simulink model "eAgriBot_V4"  (R2022b)
settings: Solver=ode3  StartTime=0.0  StopTime=t_sim  FixedStep=step_size  RelTol=1e-3
values from neighbouring files (symbols this model uses):
  accel = 0.1*9.81    (= 0.981)    [Run_eAgriBot_V4.m]
  B_tines = 5    [Run_eAgriBot_V4.m]
  brake_bias = 1    [Run_eAgriBot_V4.m]
  c = 6100    [Run_eAgriBot_V4.m]
  decel = 0.15*9.81    (= 1.4715)    [Run_eAgriBot_V4.m]
  decel_begin_dist = total_dist_target    (= 100)    [Run_eAgriBot_V4.m]
  drivetype = 3    [Run_eAgriBot_V4.m]
  effmap = [0.5 0.586 0.723 0.778 0.614 0.604 0.6 0.584 0.709 0.658 0.586 0.688 ... (121 elements, 11x11)]    [EM_effmap_generic.mat]
  end_delay = 4    [Run_eAgriBot_V4.m]
  F_tines = 5    [Run_eAgriBot_V4.m]
  Fb_max = m*g    (= 5101.2)    [Run_eAgriBot_V4.m]
  FT_c_x_rel = l_f    (= 0.645)    [Run_eAgriBot_V4.m]
  FT_c_z_rel = R_u-h_CoG    (= -0.2825)    [Run_eAgriBot_V4.m]
  g = 9.81    [Run_eAgriBot_V4.m]
  gb_eff = 0.98    [Run_eAgriBot_V4.m]
  ground_coh = c*ones(length(ground_points),1)    [Run_eAgriBot_V4.m]
  ground_dens = gamma_s*ones(length(ground_points),1)    [Run_eAgriBot_V4.m]
  ground_height = zeros(length(ground_points),1)    [Run_eAgriBot_V4.m]
  ground_kxy = k_xy*ones(length(ground_points),1)    [Run_eAgriBot_V4.m]
  ground_res = 0.01    [Run_eAgriBot_V4.m]
  Har_back_tip_x_rel = Har_back_top_x_rel+Har_tine_length*cos(Har_angle)    [Run_eAgriBot_V4.m]
  Har_back_tip_z_rel = abs(Hook_z_rel)-h_CoG-Har_tine_depth    [Run_eAgriBot_V4.m]
  Har_back_top_x_rel = -2.0    (= -2)    [Run_eAgriBot_V4.m]
  Har_back_top_z_rel = Har_back_tip_z_rel+Har_tine_length*sin(Har_angle)    [Run_eAgriBot_V4.m]
  Har_front_tip_x_rel = Har_front_top_x_rel+Har_tine_length*cos(Har_angle)    [Run_eAgriBot_V4.m]
  Har_front_tip_z_rel = abs(Hook_z_rel)-h_CoG-Har_tine_depth    [Run_eAgriBot_V4.m]
  Har_front_top_x_rel = -1.2    [Run_eAgriBot_V4.m]
  Har_front_top_z_rel = Har_front_tip_z_rel+Har_tine_length*sin(Har_angle)    [Run_eAgriBot_V4.m]
  Har_tine_length = 0.25    [Run_eAgriBot_V4.m]
  Har_tine_width = 0.02    [Run_eAgriBot_V4.m]
  Har_tire_rad = 0.5842/2    (= 0.2921)    [Run_eAgriBot_V4.m]
  Har_tire_x_rel = -1.5    [Run_eAgriBot_V4.m]
  Har_tire_z_rel = abs(Hook_z_rel)-h_CoG+Har_tire_rad    [Run_eAgriBot_V4.m]
  Hook_x_rel = l_f-l-0.4    (= -1.045)    [Run_eAgriBot_V4.m]
  Hook_z_rel = -0.3    [Run_eAgriBot_V4.m]
  i_front = 17.9542    [Run_eAgriBot_V4.m]
  I_gain = 0.0    (= 0)    [Run_eAgriBot_V4.m]
  i_rear = 17.9542    [Run_eAgriBot_V4.m]
  I_y = 150    [Run_eAgriBot_V4.m]
  I_y_tool = 20    [Run_eAgriBot_V4.m]
  index_init = round(FT_init_exit_x/ground_res)+1    [Run_eAgriBot_V4.m]
  init_CoG_height = h_CoG-0.001    (= 0.599)    [Run_eAgriBot_V4.m]
  init_CoG_v_z = 0    [Run_eAgriBot_V4.m]
  init_omega = 0    [Run_eAgriBot_V4.m]
  init_theta = 0    [Run_eAgriBot_V4.m]
  J_front = J_drive    (= 15)    [Run_eAgriBot_V4.m]
  J_harrow = 1    [Run_eAgriBot_V4.m]
  J_rear = J_drive    (= 15)    [Run_eAgriBot_V4.m]
  k_d = 50e2    (= 5000)    [Run_eAgriBot_V4.m]
  k_d_har = 50e2    (= 5000)    [Run_eAgriBot_V4.m]
  m = 520    [Run_eAgriBot_V4.m]
  m_tool = 200    [Run_eAgriBot_V4.m]
  main_cycle_delay = 5    [Run_eAgriBot_V4.m]
  mu = 0.35    [Run_eAgriBot_V4.m]
  omega_tool_init = 0    [Run_eAgriBot_V4.m]
  P_aux = 200    [Run_eAgriBot_V4.m]
  P_gain = 1.0    (= 1)    [Run_eAgriBot_V4.m]
  pack_Ah = 360    [Battery_data_V5_Kokam_NMC.mat]
  pack_R_charge = [0.00267222222222 0.00267222222222 0.00317777777778 0.00310555555556 0.0026 0.00281666666667 0.00332222222222 0.00353888888889 0.00325 0.00382777777778 0.00382777777778]    [Battery_data_V5_Kokam_NMC.mat]
  pack_R_discharge = [0.00267222222222 0.00267222222222 0.00317777777778 0.00310555555556 0.0026 0.00281666666667 0.00332222222222 0.00353888888889 0.00325 0.00382777777778 0.00382777777778]    [Battery_data_V5_Kokam_NMC.mat]
  pack_VOC = [54.509 52.351 50.895 49.556 48.477 47.645 47.008 46.449 45.825 44.941 44.941]    [Battery_data_V5_Kokam_NMC.mat]
  params2 = [exit_angle reso theta_m_max s_d_tol po]    [Run_eAgriBot_V4.m]
  phi = 26.6    [Run_eAgriBot_V4.m]
  pre_accel = 0.1*9.81    (= 0.981)    [Run_eAgriBot_V4.m]
  pre_decel = 0.15*9.81    (= 1.4715)    [Run_eAgriBot_V4.m]
  pre_decel_begin_dist = pre_dist_target-pre_decel_dist    (= 2.34454218631)    [Run_eAgriBot_V4.m]
  pre_vel = 5    [Run_eAgriBot_V4.m]
  r_front = R_u    (= 0.3175)    [Run_eAgriBot_V4.m]
  r_rear = R_u    (= 0.3175)    [Run_eAgriBot_V4.m]
  rho_t = gamma_s/9.81    (= 1664.01630989)    [Run_eAgriBot_V4.m]
  RT_c_x_rel = l_f-l    (= -0.645)    [Run_eAgriBot_V4.m]
  RT_c_z_rel = R_u-h_CoG    (= -0.2825)    [Run_eAgriBot_V4.m]
  s_init = 3    [Run_eAgriBot_V4.m]
  simu_max_time = cycle_total_time*4    (= 259.930519878)    [Run_eAgriBot_V4.m]
  slip_init = 0    [Run_eAgriBot_V4.m]
  slip_ub = r_rear*1.75    (= 0.555625)    [Run_eAgriBot_V4.m]
  slip_ub_har = Har_tire_rad*1.90    (= 0.55499)    [Run_eAgriBot_V4.m]
  SOC_init = 0.8    [Run_eAgriBot_V4.m]
  SOD = [0 0.1 0.2 0.3 0.4 0.5 0.6 0.7 0.8 0.9 1]    [Battery_data_V5_Kokam_NMC.mat]
  sr_lim_skid = -0.2    [Run_eAgriBot_V4.m]
  sr_lim_slip_f = 0.20-slip_trig    (= 0.18)    [Run_eAgriBot_V4.m]
  sr_lim_slip_r = 0.14-slip_trig    (= 0.12)    [Run_eAgriBot_V4.m]
  step_size = 1e-3    (= 0.001)    [Run_eAgriBot_V4.m]
  T = [80 80 75 70.5882352941 66.6666666667 63.1578947368 60 57.1428571429 54.5454545455 52.1739130435 50 48 ... (49 elements, 49x1)]    [EM_data_V4.mat]    (also in Run_eAgriBot_V4.m = 2*T)
  T_effmap = [0 8 16 24 32 40 48 56 64 72 80]    [EM_effmap_generic.mat]    (also in Run_eAgriBot_V4.m = 2*T_effmap)
  T_multi_r = 1.5    [Run_eAgriBot_V4.m]
  t_params = [c k_c k_phi phi k_xy gamma_s R_u wid c_0 c_1 c_0f c_1f n_0 n_1 k_1 k_2 k_3]    [Run_eAgriBot_V4.m]
  t_params_har = [c k_c k_phi phi k_xy gamma_s Har_tire_rad Har_tire_wid c_0 c_1 c_0f c_1f n_0 n_1 k_1 k_2 k_3]    [Run_eAgriBot_V4.m]
  theta_tool_init = 0    [Run_eAgriBot_V4.m]
  Tine_vz_damping = 0    [Run_eAgriBot_V4.m]
  Tool_x_rel = -1.3    [Run_eAgriBot_V4.m]
  Tool_z_rel = -0.08    [Run_eAgriBot_V4.m]
  v_init = 0    [Run_eAgriBot_V4.m]
  vel_max = 8    [Run_eAgriBot_V4.m]
  w = [0 75 80 85 90 95 100 105 110 115 120 125 ... (49 elements, 49x1)]    [EM_data_V4.mat]
  w_effmap = [0 31.4159265359 62.8318530718 94.2477796077 125.663706144 157.079632679 188.495559215 219.911485751 251.327412287 282.743338823 314.159265359]    [EM_effmap_generic.mat]
libraries: slpidlib x1, simulink x1
(part 3 of 4)

== system eAgriBot_V4/Vehicle dynamics/Towed tool calculations/Vertical force damping ==
  Har_tire_z : Inport
  Har_tire_vz : Inport  Port=2
  F_sigma_zhar : Inport  Port=3
  F_tau_zhar : Inport  Port=4
  Abs : Abs  SaturateOnIntegerOverflow=off
  Abs1 : Abs  SaturateOnIntegerOverflow=off
  Constant2 : Constant  Value=0
  Constant3 : Constant  Value=0
  Constant4 : Constant  Value=0
  Divide : Product  Inputs=*/
  Divide1 : Product  Inputs=*/
  Gain2 : Gain  Gain=k_d_har
  Product : Product
  Product1 : Product
  Sum1 : Sum  Inputs=|+-
  Sum2 : Sum  Inputs=|++
  Sum3 : Sum  Inputs=|++
  Sum4 : Sum  Inputs=-+|
  Sum5 : Sum  Inputs=|++
  Switch2 : Switch  Criteria=u2 > Threshold  SaturateOnIntegerOverflow=off  InputSameDT=off
  Switch3 : Switch  Criteria=u2 ~= 0  SaturateOnIntegerOverflow=off  InputSameDT=off
  Switch4 : Switch  Criteria=u2 ~= 0  SaturateOnIntegerOverflow=off  InputSameDT=off
  To Workspace1 : ToWorkspace  VariableName=Fz_har  SaveFormat=Timeseries  SampleTime=-1
  F_sigma_zhar_d : Outport
  F_tau_zhar_d : Outport  Port=2
  wires:
  Sum1/1 -> Sum5/1, F_sigma_zhar_d/1
  Har_tire_vz/1 -> Gain2/1
  Gain2/1 -> Switch2/3
  Har_tire_z/1 -> Switch2/2
  Switch2/1 -> Product1/1, Product/1
  Constant2/1 -> Switch2/1
  Sum2/1 -> Divide/2, Switch3/2
  Constant3/1 -> Switch3/3
  Divide/1 -> Abs/1
  Abs/1 -> Switch3/1
  Switch3/1 -> Product/2
  Product/1 -> Sum1/2
  Sum3/1 -> Divide1/2, Switch4/2
  Abs1/1 -> Switch4/1
  Constant4/1 -> Switch4/3
  F_tau_zhar/1 -> Sum4/2, Sum3/1, Divide1/1, Sum2/2
  Divide1/1 -> Abs1/1
  F_sigma_zhar/1 -> Sum2/1, Sum3/2, Sum1/1, Divide/1
  Switch4/1 -> Product1/2
  Product1/1 -> Sum4/1
  Sum4/1 -> Sum5/2, F_tau_zhar_d/1
  Sum5/1 -> To Workspace1/1

== system eAgriBot_V4/Vehicle dynamics/Towed tool calculations/Vertical force damping1 ==
  Har_tire_z : Inport
  Har_tire_vz : Inport  Port=2
  F_sigma_zhar : Inport  Port=3
  Constant2 : Constant  Value=0
  Gain2 : Gain  Gain=k_d_har
  Sum1 : Sum  Inputs=|+-
  Switch2 : Switch  Criteria=u2 > Threshold  SaturateOnIntegerOverflow=off  InputSameDT=off
  F_sigma_zhar_d : Outport
  wires:
  Sum1/1 -> F_sigma_zhar_d/1
  Har_tire_vz/1 -> Gain2/1
  Gain2/1 -> Switch2/3
  Har_tire_z/1 -> Switch2/2
  Switch2/1 -> Sum1/2
  Constant2/1 -> Switch2/1
  F_sigma_zhar/1 -> Sum1/1

== matlab function eAgriBot_V4/Vehicle dynamics/Position and velocity of the wheels (output values are for wheel bottom points)/MATLAB Function ==
  data: theta input; RT_x output; RT_z output; FT_x output; FT_z output; RT_vx output; RT_vz output; FT_vx output; FT_vz output; omega input; CoG_vx input; CoG_x input; CoG_vz input; CoG_z input; RT_c_z_rel input; RT_c_x_rel input; FT_c_z_rel input; FT_c_x_rel input; r_rear input; r_front input
function [RT_x, RT_z, FT_x, FT_z, RT_vx, RT_vz, FT_vx, FT_vz] =...
    fcn(theta, omega, CoG_vx, CoG_x, CoG_vz, CoG_z, RT_c_z_rel,...
    RT_c_x_rel, FT_c_z_rel, FT_c_x_rel, r_rear, r_front)

    % theta: Vehicle pitch
    % omega: Vehicle pitch rate
    % CoG_x: Current x-position of the CoG
    % CoG_z: Current z-position of the CoG
    % RT/FT_c_z_rel: Difference between rear/front tire z-coordinate and the CoG
    % z-coordinate when pitch is zero.
    % RT/FT_c_x_rel: Difference between rear/front tire x-coordinate and the CoG
    % x-coordinate when pitch is zero.
    % r_rear: Rear tire radius
    % r_front: Front tire radius
    
    RT_center = [cos(theta) sin(theta); -sin(theta) cos(theta)]*...
        [RT_c_x_rel; RT_c_z_rel]+[CoG_x; CoG_z];
    
    RT_x = RT_center(1);
    RT_z = RT_center(2)-r_rear;
    
    FT_center = [cos(theta) sin(theta); -sin(theta) cos(theta)]*...
        [FT_c_x_rel; FT_c_z_rel]+[CoG_x; CoG_z];
    
    FT_x = FT_center(1);
    FT_z = FT_center(2)-r_front;
    
    RT_vec_x = RT_x-CoG_x;
    RT_vec_z = RT_z-CoG_z;
    RT_vec = [RT_vec_x; 0; RT_vec_z];
    
    RT_vel = [CoG_vx; 0; CoG_vz]+cross([0; omega; 0], RT_vec);
    RT_vx = RT_vel(1);
    RT_vz = RT_vel(3);
    
    FT_vec_x = FT_x-CoG_x;
    FT_vec_z = FT_z-CoG_z;
    FT_vec = [FT_vec_x; 0; FT_vec_z];
    
    FT_vel = [CoG_vx; 0; CoG_vz]+cross([0; omega; 0], FT_vec);
    FT_vx = FT_vel(1);
    FT_vz = FT_vel(3);

end

== matlab function eAgriBot_V4/Vehicle dynamics/Ground properties update for rear tire/MATLAB Function ==
  data: index_upd_high output; index_upd_low output; t_params input; ground_res input; ground_height output; dens output; coh output; kx output; params2 input; FT_x input; FT_z input; sr_f input; ground_height input; dens input; coh input; kx input; prev_index input; index output
function [index_upd_high, index_upd_low, ground_height, dens, coh, kx, index]= fcn(t_params, ground_res, params2,...
    FT_x, FT_z, sr_f, ground_height, dens, coh, kx, prev_index)

    R_u = t_params(7);
    ea = deg2rad(params2(1));
    c = t_params(1);
    gamma_s = t_params(6);
    k_x = t_params(5);
    k_1 = t_params(15);
    k_2 = t_params(16);
    k_3 = t_params(17);

    n_p = 1;

    FT_exit_x = FT_x+R_u*sin(ea);
    FT_exit_z = FT_z+(R_u-R_u*cos(ea));

    FT_exit_dens = gamma_s*(1+(1-exp(-abs(sr_f)/k_1))*k_2+k_3*n_p);
    FT_exit_coh = c*(1+(1-exp(-abs(sr_f)/k_1))*k_2+k_3*n_p);
    FT_exit_kx = k_x*(1-(1-exp(-abs(sr_f)/k_1))*k_2-k_3*n_p);

    index = round(FT_exit_x/ground_res)+1;

    ground_height(index,1) = FT_exit_z;

    dens(index,1) = FT_exit_dens;

    coh(index,1) = FT_exit_coh;

    kx(index,1) = FT_exit_kx;
    
    % index_upd_high and index_upd_low are needed for updating the soil
    % values for the harrow tines
    index_upd_high = index;
    index_upd_low = index;


    if index > (prev_index+1)
        num_points_tofix = index-(prev_index+1);
        index_upd_low = prev_index+1;
        for i = 1:num_points_tofix
            ground_height(prev_index+i,1) = (ground_height(index,1)-ground_height(prev_index,1))*...
                i/(num_points_tofix+1)+ground_height(prev_index,1);

            dens(prev_index+i,1) = (dens(index,1)-dens(prev_index,1))*...
                i/(num_points_tofix+1)+dens(prev_index,1);

            coh(prev_index+i,1) = (coh(index,1)-coh(prev_index,1))*...
                i/(num_points_tofix+1)+coh(prev_index,1);

            kx(prev_index+i,1) = (kx(index,1)-kx(prev_index,1))*...
                i/(num_points_tofix+1)+kx(prev_index,1);
        end
    end

end

== matlab function eAgriBot_V4/Vehicle dynamics/Ground properties update for rear tire/MATLAB Function1 ==
  data: RT_x input; RT_z input; ground_height input; dens input; coh input; kx input; ground_res input; t_params input; upd_RT_z output; upd_dens output; upd_coh output; upd_kx output
function [upd_RT_z, upd_dens, upd_coh, upd_kx] = fcn(RT_x, RT_z, ground_height, dens, coh, kx, ground_res, t_params)

    
    R_u = t_params(7);
    ind_L = max(round((RT_x-R_u)/ground_res)+1, 1);
    ind_R = max(round((RT_x+R_u)/ground_res)+1, 1);

    upd_RT_z = RT_z-mean(ground_height(ind_L:ind_R));
    upd_dens = mean(dens(ind_L:ind_R));
    upd_coh = mean(coh(ind_L:ind_R));
    upd_kx = mean(kx(ind_L:ind_R));

end

== matlab function eAgriBot_V4/Vehicle dynamics/Towed tool calculations/Tool position, velocity, and acceleration calc/Tool position, velocity, and acceleration calc ==
  data: alpha input; omega input; theta input; Hook_x output; CoG_x input; CoG_z input; CoG_v_x input; CoG_v_z input; CoG_a_x input; CoG_a_z input; alpha_tool input; omega_tool input; theta_tool input; Hook_x_rel input; Hook_z_rel input; Hook_z output; Hook_v_x output; Hook_v_z output; Hook_a_x output; Hook_a_z output; Tool_CoG_x output; Tool_CoG_z output; Tool_CoG_a_x output; Tool_CoG_a_z output; Tool_x_rel input; Tool_z_rel input; Har_back_top_x_rel input; Har_back_top_z_rel input; Har_back_tip_x_rel input; Har_back_tip_z_rel input; Har_front_top_x_rel input; Har_front_top_z_rel input; Har_front_tip_x_rel input; Har_front_tip_z_rel input; Har_tire_x_rel input; Har_tire_z_rel input; Har_tire_radius input; Harrow_back_mid_x output; Harrow_back_mid_z output; Harrow_back_tip_z output; Harrow_back_mid_v_x output; Harrow_back_mid_v_z output; Harrow_front_mid_x output; Harrow_front_mid_z output; Harrow_front_tip_z output; Harrow_front_mid_v_x output; Harrow_front_mid_v_z output; Harrow_tire_bottom_x output; Harrow_tire_bottom_z output; Harrow_tire_bottom_v_x output; Harrow_tire_bottom_v_z output; Harrow_back_angle output; Harrow_front_angle output; Harrow_front_tip_x output; Harrow_back_tip_x output
function [Hook_x, Hook_z, Hook_v_x, Hook_v_z, Hook_a_x, Hook_a_z,...
    Tool_CoG_x, Tool_CoG_z, Tool_CoG_a_x, Tool_CoG_a_z,...
    Harrow_back_mid_x,...
    Harrow_back_mid_z, Harrow_back_tip_z, Harrow_back_mid_v_x,...
    Harrow_back_mid_v_z, Harrow_front_mid_x, Harrow_front_mid_z,...
    Harrow_front_tip_z, Harrow_front_mid_v_x, Harrow_front_mid_v_z,...
    Harrow_tire_bottom_x, Harrow_tire_bottom_z, Harrow_tire_bottom_v_x,...
    Harrow_tire_bottom_v_z, Harrow_back_angle, Harrow_front_angle, Harrow_front_tip_x,...
    Harrow_back_tip_x] = fcn(alpha,...
    omega, theta, CoG_x, CoG_z, CoG_v_x, CoG_v_z, CoG_a_x, CoG_a_z, alpha_tool,...
    omega_tool, theta_tool, Hook_x_rel, Hook_z_rel, Tool_x_rel, Tool_z_rel,...
    Har_back_top_x_rel, Har_back_top_z_rel,...
    Har_back_tip_x_rel, Har_back_tip_z_rel, Har_front_top_x_rel, Har_front_top_z_rel,...
    Har_front_tip_x_rel, Har_front_tip_z_rel, Har_tire_x_rel, Har_tire_z_rel, Har_tire_radius)

    % Calculate the current position of the hook

    % Hook_x_rel and Hook_z_rel describe the position of the hook in
    % relation to the CoG of the vehicle when the vehicle is on flat
    % ground.
    Hook_pos = [cos(theta) sin(theta); -sin(theta) cos(theta)]*...
            [Hook_x_rel; Hook_z_rel]+[CoG_x; CoG_z];
    
    Hook_x = Hook_pos(1);
    Hook_z = Hook_pos(2);

    % Calculate the current velocity of the hook
    vec_CoG_hook = [Hook_x-CoG_x; 0; Hook_z-CoG_z];
    Hook_v = [CoG_v_x; 0; CoG_v_z] + cross([0; omega; 0], vec_CoG_hook);

    Hook_v_x = Hook_v(1);
    Hook_v_z = Hook_v(3);

    % Calculate the current acceleration of the hook

    alpha_2 = [0; alpha; 0];
    omega_2 = [0; omega; 0];

    Hook_a = [CoG_a_x; 0; CoG_a_z] + cross(alpha_2, vec_CoG_hook) + cross(omega_2, cross(omega_2, vec_CoG_hook));

    Hook_a_x = Hook_a(1);
    Hook_a_z = Hook_a(3);

    % Calculate the current acceleration of the CoG of the tool

    % Tool_x_rel and Tool_z_rel describe the position of the tool CoG in
    % relation to the hook when the vehicle is on flat
    % ground.
    Tool_CoG_pos = [cos(theta_tool) sin(theta_tool); -sin(theta_tool) cos(theta_tool)]*...
            [Tool_x_rel; Tool_z_rel]+[Hook_x; Hook_z];

    Tool_CoG_x = Tool_CoG_pos(1);
    Tool_CoG_z = Tool_CoG_pos(2);

    vec_toolCoG_hook = [Hook_x-Tool_CoG_x; 0; Hook_z-Tool_CoG_z];

    alpha_tool_2 = [0; alpha_tool; 0];
    omega_tool_2 = [0; omega_tool; 0];

    Tool_CoG_a = Hook_a - cross(alpha_tool_2,vec_toolCoG_hook) - cross(omega_tool_2, cross(omega_tool_2,vec_toolCoG_hook));

    Tool_CoG_a_x = Tool_CoG_a(1);
    Tool_CoG_a_z = Tool_CoG_a(3);

    % Calculate the current position and velocity of the bottom point of
    % the tool.

    % Tool_bottom_x_rel and Tool_bottom_z_rel describe the position of the
    % bottom point of the tool in relation to the hook when the vehicle and
    % tool are on flat ground.

    % New stuff, harrow

    Harrow_back_top_pos = [cos(theta_tool) sin(theta_tool); -sin(theta_tool) cos(theta_tool)]*...
        [Har_back_top_x_rel; Har_back_top_z_rel]+[Hook_x; Hook_z];
    
    Harrow_back_tip_pos = [cos(theta_tool) sin(theta_tool); -sin(theta_tool) cos(theta_tool)]*...
        [Har_back_tip_x_rel; Har_back_tip_z_rel]+[Hook_x; Hook_z];

    Harrow_back_tip_x = Harrow_back_tip_pos(1);
    Harrow_back_tip_z = Harrow_back_tip_pos(2);

    Harrow_front_top_pos = [cos(theta_tool) sin(theta_tool); -sin(theta_tool) cos(theta_tool)]*...
        [Har_front_top_x_rel; Har_front_top_z_rel]+[Hook_x; Hook_z];

    Harrow_front_tip_pos = [cos(theta_tool) sin(theta_tool); -sin(theta_tool) cos(theta_tool)]*...
        [Har_front_tip_x_rel; Har_front_tip_z_rel]+[Hook_x; Hook_z];

    Harrow_front_tip_x = Harrow_front_tip_pos(1);
    Harrow_front_tip_z = Harrow_front_tip_pos(2);

    % Back row
    
    if Harrow_back_top_pos(2) >= 0
        Harrow_back_mid_z = Harrow_back_tip_pos(2)/2;
        % Calculate gradient and constant (c) in line equation
        Harrow_back_grad = (Harrow_back_tip_pos(2)-Harrow_back_top_pos(2))/(Harrow_back_tip_pos(1)-Harrow_back_top_pos(1));
        Harrow_back_c = Harrow_back_tip_pos(2)-Harrow_back_tip_pos(1)*Harrow_back_grad;
        % Calculate mid point of the tine
        Harrow_back_mid_x = (Harrow_back_mid_z-Harrow_back_c)/Harrow_back_grad;
    else
        Harrow_back_mid_z = (Harrow_back_tip_pos(2)+Harrow_back_top_pos(2))/2;
        Harrow_back_mid_x = (Harrow_back_tip_pos(1)+Harrow_back_top_pos(1))/2;
    end
    Harrow_back_angle = -1*asin((Harrow_back_tip_pos(2)-Harrow_back_top_pos(2))/(Harrow_back_tip_pos(1)-Harrow_back_top_pos(1)));
    Harrow_back_depth = Harrow_back_tip_pos(2);

    vec_Hook_backtip = [Harrow_back_tip_pos(1)-Hook_x; 0; Harrow_back_tip_pos(2)-Hook_z];
    Harrow_back_mid_v = [Hook_v_x; 0; Hook_v_z] + cross([0; omega_tool; 0], vec_Hook_backtip);

    Harrow_back_mid_v_x = Harrow_back_mid_v(1);
    Harrow_back_mid_v_z = Harrow_back_mid_v(3);

    % Front row
    
    if Harrow_front_top_pos(2) >= 0
        Harrow_front_mid_z = Harrow_front_tip_pos(2)/2;
        % Calculate gradient and constant (c) in line equation
        Harrow_front_grad = (Harrow_front_tip_pos(2)-Harrow_front_top_pos(2))/(Harrow_front_tip_pos(1)-Harrow_front_top_pos(1));
        Harrow_front_c = Harrow_front_tip_pos(2)-Harrow_front_tip_pos(1)*Harrow_front_grad;
        % Calculate mid point of the tine
        Harrow_front_mid_x = (Harrow_front_mid_z-Harrow_front_c)/Harrow_front_grad;
    else
        Harrow_front_mid_z = (Harrow_front_tip_pos(2)+Harrow_front_top_pos(2))/2;
        Harrow_front_mid_x = (Harrow_front_tip_pos(1)+Harrow_front_top_pos(1))/2;
    end
    Harrow_front_angle = -1*asin((Harrow_front_tip_pos(2)-Harrow_front_top_pos(2))/(Harrow_front_tip_pos(1)-Harrow_front_top_pos(1)));
    Harrow_front_depth = Harrow_front_tip_pos(2);

    vec_Hook_fronttip = [Harrow_front_tip_pos(1)-Hook_x; 0; Harrow_front_tip_pos(2)-Hook_z];
    Harrow_front_mid_v = [Hook_v_x; 0; Hook_v_z] + cross([0; omega_tool; 0], vec_Hook_fronttip);

    Harrow_front_mid_v_x = Harrow_front_mid_v(1);
    Harrow_front_mid_v_z = Harrow_front_mid_v(3);

    Harrow_tire_pos = [cos(theta_tool) sin(theta_tool); -sin(theta_tool) cos(theta_tool)]*...
        [Har_tire_x_rel; Har_tire_z_rel]+[Hook_x; Hook_z];

    Harrow_tire_bottom_x = Harrow_tire_pos(1);
    Harrow_tire_bottom_z = Harrow_tire_pos(2)-Har_tire_radius;
    
    vec_Hook_tirebottom = [Harrow_tire_bottom_x-Hook_x; 0; Harrow_tire_bottom_z-Hook_z];
    Harrow_tire_bottom_v = [Hook_v_x; 0; Hook_v_z] + cross([0; omega_tool; 0], vec_Hook_tirebottom);

    Harrow_tire_bottom_v_x = Harrow_tire_bottom_v(1);
    Harrow_tire_bottom_v_z = Harrow_tire_bottom_v(3);

    % Needs to output:
    % Harrow_back_mid_x, Harrow_back_mid_z, Harrow_back_tip_z
    % Harrow_back_mid_v_x, Harrow_back_mid_v_z
    % Harrow_front_mid_x, Harrow_front_mid_z, Harrow_front_tip_z
    % Harrow_front_mid_v_x, Harrow_front_mid_v_z
    % Harrow_tire_bottom_x, Harrow_tire_bottom_z
    % Harrow_tire_bottom_v_x, Harrow_tire_bottom_v_z

    % Needs as inputs:
    % Har_back_top_x_rel, Har_back_top_z_rel
    % Har_back_tip_x_rel, Har_back_tip_z_rel
    % Har_front_top_x_rel, Har_front_top_z_rel
    % Har_front_tip_x_rel, Har_front_tip_z_rel
    % Har_tire_x_rel, Har_tire_z_rel, Har_tire_radius

end

== matlab function eAgriBot_V4/Tire model (FRONT)/slip_ratio calc ==
  data: r_front input; v_ms input; FT_vx input; w_tire input; sr output; slip_ub input
function sr = fcn(r_front, v_ms, FT_vx, w_tire, slip_ub)
    
    ub = slip_ub; % upper bound (when the rotational speed is 1 rad/s)
    lb = 0.1/3.6; % lower bound

    v_ms = max(0, v_ms);

    if abs(v_ms) > ub
        sr = (w_tire*r_front-FT_vx)/FT_vx;
    elseif abs(v_ms) < lb
        sr = w_tire*r_front-FT_vx;
    elseif abs(v_ms) <= ub && abs(v_ms) >= lb
        sr = (1/(ub-lb))*(ub-v_ms)*(w_tire*r_front-FT_vx)+(1/(ub-lb))*(v_ms-lb)*((w_tire*r_front-FT_vx)/FT_vx);
    else
        sr = 0;
    end
    
    sr = max(-1, sr);

end

== matlab function eAgriBot_V4/Tire model (REAR)/Tire force calc1 ==
  data: T output; v_ms input; w_tire_pure input; s_d input; t_params input; params2 input; h input; gamma_s input; c input; k_xy input; F_sigma_z output; F_sigma_x output; F_sigma_angle output; F_tau_z output; F_tau_x output; F_tau_angle output; drivetype input
function [T, F_sigma_z, F_sigma_x, F_sigma_angle, F_tau_z, F_tau_x, F_tau_angle]  = fcn(v_ms, w_tire_pure, s_d, t_params, params2, h, gamma_s, c, k_xy, drivetype)

    %%

% function [W, F_x, T] = ReeceFuncSim_V1(s_d, h, t_params, params2)
%     c = t_params(1); % Pa
    k_c = t_params(2); % 34 default
    k_phi = t_params(3); % 49.68 default
    % n = 0.7;
    phi = t_params(4); % deg
%     k_xy = t_params(5); % m
%     gamma_s = t_params(6); % N/m^3
    
    R_u = t_params(7); % m (tire radius)
    w = t_params(8); % m (tire width)
    c_0 = t_params(9);
    c_1 = t_params(10);
    c_0f = t_params(11);
    c_1f = t_params(12);
    n_0 = t_params(13);
    n_1 = t_params(14);
    k_1 = t_params(15);
    k_2 = t_params(16);
    k_3 = t_params(17);

%     h = RT_upd_params(1);
%     gamma_s = RT_upd_params(2);
%     c = RT_upd_params(3);
%     k_xy = RT_upd_params(4);
    
    exit_angle = params2(1);
    reso = params2(2); % Angle resolution, number of segments per one degree
    
    theta_m_max = params2(3); % Maximum percentage of theta_e allowed for theta_m
    % Allowing this to go too high may result in issues with some
    % calculations outputting complex numbers.
    
    s_d_tol = params2(4);
    
    po = params2(5);
    
    if h < 0
        % Start with defining the angles for theta
        % Then calculate the different values, e.g., sigma_n
        % for each angle.
        % The angle theta starts counter-clockwise from the
        % bottom of the tire (page 3 (267))
        theta_e = min(acos((R_u+max(h,-R_u))/R_u), deg2rad(89));
        theta_b = deg2rad(exit_angle);
        if s_d < -1*s_d_tol
            a = 1/(1+abs(s_d));
        
            d = tan(deg2rad(45)-deg2rad(phi/2));
            
            theta_m = min(2*atan(d./(-a-1)+sqrt(d^2./(-a-1).^2-(-a+1)./(-a-1))), theta_m_max*theta_e);
        elseif s_d >= -1*s_d_tol && s_d <= 0
            a = 1/(1+abs(s_d));
            d = tan(deg2rad(45)-deg2rad(phi/2));
            tm1 = min(2*atan(d./(-a-1)+sqrt(d^2./(-a-1).^2-(-a+1)./(-a-1))), theta_m_max*theta_e);
            tm2 = min((c_0+c_1*abs(s_d)), theta_m_max)*theta_e;
            ft = (1/(s_d_tol)*s_d+1)^po;
            theta_m = (1-ft)*tm1+ft*tm2;
        else
            theta_m = min((c_0+c_1*abs(s_d)), theta_m_max)*theta_e;
        end
        
        angles = linspace(theta_b,theta_e,ceil(rad2deg(theta_e-theta_b)*reso));
        
        l_p = (theta_e-theta_b)*R_u; % Contact arc length
        n = n_0+n_1*abs(s_d);
        b = min(w, l_p);
        
        sigma_n = zeros(length(angles),1);
        W_dtheta = zeros(length(angles),1);
        tau_max = zeros(length(angles),1);
        tau_x = zeros(length(angles),1);
        F_x_dtheta = zeros(length(angles),1);
        T_dtheta = zeros(length(angles),1);
        j_x = zeros(length(angles),1);
        K_v = zeros(length(angles),1);

        F_sigma_dx = zeros(length(angles),1);
        F_sigma_dz = zeros(length(angles),1);
        F_tau_dx = zeros(length(angles),1);
        F_tau_dz = zeros(length(angles),1);

        sigma_theta = zeros(length(angles),1);
        tau_theta = zeros(length(angles),1);
        
        for i = 1:length(angles)
            if angles(i) >= theta_m
                sigma_n(i,1) = (c*k_c+b*gamma_s*k_phi)*(R_u/b)^n*(cos(angles(i))-cos(theta_e))^n;
            else
                sigma_n(i,1) = (c*k_c+b*gamma_s*k_phi)*(R_u/b)^n...
                    *(cos(theta_e-((angles(i)-theta_b)/(theta_m-theta_b)*(theta_e-theta_m)))-cos(theta_e))^n;
            end

            sigma_theta(i,1) = angles(i)*sigma_n(i,1);
        
            tau_max(i,1) = c+sigma_n(i,1)*tan(deg2rad(phi));
        
            if s_d > 0
                j_x(i,1) = R_u*((theta_e-angles(i))-(1-s_d)*(sin(theta_e)-sin(angles(i))));
            elseif s_d >= -1*s_d_tol && s_d <= 0
                j_x1 = R_u*((theta_e-angles(i))-(1-s_d)*(sin(theta_e)-sin(angles(i))));
                a = 1/(1+abs(s_d));
                K_v(i,1) = a*(((1+abs(s_d))*(sin(theta_e)-sin(theta_m)))/(theta_e-theta_m)-1);
                if angles(i) >= theta_m
                    j_x2 = R_u*((theta_e-angles(i))*(1+K_v(i,1)*(1+abs(s_d)))-(1+abs(s_d))*(sin(theta_e)-sin(angles(i))));
                else
                    j_x2 = R_u*((theta_m-angles(i))-(1+abs(s_d))*(sin(theta_m)-sin(angles(i))));
                end
                ft = (1/(s_d_tol)*s_d+1)^po;
                j_x(i,1) = (1-ft)*j_x2+ft*j_x1;
            else
                a = 1/(1+abs(s_d));
                K_v(i,1) = a*(((1+abs(s_d))*(sin(theta_e)-sin(theta_m)))/(theta_e-theta_m)-1);
                if angles(i) >= theta_m
                    j_x(i,1) = R_u*((theta_e-angles(i))*(1+K_v(i,1)*(1+abs(s_d)))-(1+abs(s_d))*(sin(theta_e)-sin(angles(i))));
                else
                    j_x(i,1) = R_u*((theta_m-angles(i))-(1+abs(s_d))*(sin(theta_m)-sin(angles(i))));
                end
            end
        end
        
        for ii = 1:length(angles)
        
            tau_x(ii,1) = max(min(tau_max(ii,1)*(1-exp(-j_x(ii,1)/k_xy)), abs(tau_max(ii,1))), -1*abs(tau_max(ii,1)));
            tau_theta(ii,1) = angles(ii)*tau_x(ii,1);

            W_dtheta(ii,1) = R_u*(sigma_n(ii,1)*cos(angles(ii))+tau_x(ii,1)*sin(angles(ii)));
            F_x_dtheta(ii,1) = R_u*(tau_x(ii,1)*cos(angles(ii))-sigma_n(ii,1)*sin(angles(ii)));
            T_dtheta(ii, 1) = R_u^2*tau_x(ii,1);

            F_sigma_dz(ii,1) = R_u*sigma_n(ii,1)*cos(angles(ii));
            F_sigma_dx(ii,1) = -1*R_u*sigma_n(ii,1)*sin(angles(ii));

            F_tau_dz(ii,1) = R_u*tau_x(ii,1)*sin(angles(ii));
            F_tau_dx(ii,1) = R_u*tau_x(ii,1)*cos(angles(ii));
        end
        
%             W = w*trapz(angles, W_dtheta);
%             F_x = w*trapz(angles, F_x_dtheta);
            T = w*trapz(angles, T_dtheta);

            F_sigma_z = w*trapz(angles, F_sigma_dz);
            F_sigma_x = w*trapz(angles, F_sigma_dx);
            F_sigma_angle = atan(-1*F_sigma_x/F_sigma_z);
            F_tau_z = w*trapz(angles, F_tau_dz);
            F_tau_x = w*trapz(angles, F_tau_dx);
            F_tau_angle = atan(F_tau_z/F_tau_x);

            F_sigma_angle = max(theta_b, min(theta_e, F_sigma_angle));
            F_tau_angle = max(theta_b, min(theta_e, F_tau_angle));

            if v_ms < 0.3/3.6
                F_sigma_angle = max(0, v_ms)*F_sigma_angle*3.6/0.3;
                F_tau_angle = max(0, v_ms)*F_tau_angle*3.6/0.3;
            end
    else
%         W = 0;
%         F_x = 0;
        T = 0;

        F_sigma_z = 0;
        F_sigma_x = 0;
        F_sigma_angle = 0;
        F_tau_z = 0;
        F_tau_x = 0;
        F_tau_angle = 0;
    end

    %%
    
%     if v_ms <= v_low/3.6
%         F_t = (T_axle-J*a_ms/R_u)/R_u;
%         F_t_res = (T_axle-J*a_ms/R_u)/R_u;
%         P = P_lim;
%     elseif (v_ms > v_low/3.6) && (v_up <= 1/3.6)
%     %          F_t = 3.6*(1/(v_up-v_low))*(v_up/3.6-v_ms)*(T_axle-J*a_ms/r)/r+3.6*(1/(v_up-v_low))*(v_ms-v_low/3.6)*(F_z*mu-F_rr);
%          F_t = 3.6*(1/(v_up-v_low))*(v_up/3.6-v_ms)*(T_axle-J*a_ms/R_u)/R_u+3.6*(1/(v_up-v_low))*(v_ms-v_low/3.6)*(F_x);
%          F_t_res = 3.6*(1/(v_up-v_low))*(v_up/3.6-v_ms)*(T_axle-J*a_ms/R_u)/R_u+3.6*(1/(v_up-v_low))*(v_ms-v_low/3.6)*(T/R_u);
%          P = 3.6*(1/(v_up-v_low))*(v_up/3.6-v_ms)*P_lim;
%     else
%         F_t = F_x;
%         F_t_res = T/R_u;
%         P = 0;
%     end

%     F_t = F_x;
    if (w_tire_pure <= 0) && (v_ms <= 0)
%         F_t = 0;
        F_sigma_x = 0;
        F_tau_x = 0;
    end
%     if v_ms <= 0
% %         F_t = max(0, F_t);
%         F_sigma_x = max(0, F_sigma_x);
%         F_tau_x = max(0, F_tau_x);
%     end
    if w_tire_pure <= 0
%         F_t = min(0, F_t);
        F_sigma_x = min(0, F_sigma_x);
%         F_tau_x = min(0, F_tau_x);
    end
%     F_t_res = T/R_u;
%     P = 0;
%     P = min(max(P, 0), P_lim);
%     T_Ft_res = F_t_res*R_u+P*(w_tire-v_ms/R_u);
%     T_Ft = F_t*R_u;

    if v_ms < 0
%         F_sigma_x = max(100*abs(v_ms), F_sigma_x);
        F_tau_x = max(500*abs(v_ms), F_tau_x);
    end

    if drivetype == 2
        F_sigma_x = F_sigma_x*abs(tanh(20*v_ms));
        F_tau_x = F_tau_x*abs(tanh(20*v_ms));
    end

    if v_ms >= 0 && v_ms < 0.1/3.6 && w_tire_pure <= 0
%         F_tau_x = F_tau_x-1e5*v_ms;
        F_tau_x = -1e1*tanh(50*v_ms);
        F_sigma_x = 0;
    end

end

== matlab function eAgriBot_V4/Vehicle dynamics/Towed tool calculations/Tine forces/Back row ==
  data: phi input; tine_length input; tine_width input; rho_t input; mu input; c input; F_x output; angle input; tine_v_x input; depth input; F_z output; g input; B_tines input; h_upd input; coh_upd input
function [F_x, F_z] = fcn(phi, tine_length, tine_width, rho_t, mu, c, angle, tine_v_x, depth, g, B_tines, h_upd, coh_upd)

L_0 = tine_length;
b = tine_width;
alpha = rad2deg(angle);
t = -1*depth;
v = tine_v_x;

if t >= 0
    gamma = (90-phi)/2;
    t_e = t*sin(deg2rad(alpha+gamma))/sin(deg2rad(gamma));
    L_1 = t*cos(deg2rad(alpha+gamma))/sin(deg2rad(gamma));
    L_2 = t_e*tan(deg2rad(alpha));
    m = rho_t*t_e*b*(L_0+(L_1+L_2)/2);
    Z = (cos(deg2rad(gamma))-tan(deg2rad(phi))*sin(deg2rad(gamma)))/(sin(deg2rad(gamma))+tan(deg2rad(phi))*cos(deg2rad(gamma)))+...
        (cos(deg2rad(alpha))-mu*sin(deg2rad(alpha)))/(sin(deg2rad(alpha))+mu*cos(deg2rad(alpha)));
    F_c = c*b*t/sin(deg2rad(gamma));
    F_a = rho_t*b*t*v^2*sin(deg2rad(alpha))/sin(deg2rad(alpha+gamma));
    F_x = m*g/Z+(F_a+F_c)/(Z*(sin(deg2rad(gamma))+tan(deg2rad(phi))*cos(deg2rad(gamma))));
    F_z = F_x*(cos(deg2rad(alpha))-mu*sin(deg2rad(alpha)))/(sin(deg2rad(alpha))+mu*cos(deg2rad(alpha)));
else
    F_x = 0;
    F_z = 0;
end

% One tine is in the ruts left by the robot tires
t_upd = h_upd*(-1);
if t_upd >= 0
    gamma = (90-phi)/2;
    t_e_upd = t_upd*sin(deg2rad(alpha+gamma))/sin(deg2rad(gamma));
    L_1_upd = t_upd*cos(deg2rad(alpha+gamma))/sin(deg2rad(gamma));
    L_2_upd = t_e_upd*tan(deg2rad(alpha));
    m = rho_t*t_e_upd*b*(L_0+(L_1_upd+L_2_upd)/2);
    Z_upd = (cos(deg2rad(gamma))-tan(deg2rad(phi))*sin(deg2rad(gamma)))/(sin(deg2rad(gamma))+tan(deg2rad(phi))*cos(deg2rad(gamma)))+...
        (cos(deg2rad(alpha))-mu*sin(deg2rad(alpha)))/(sin(deg2rad(alpha))+mu*cos(deg2rad(alpha)));
    F_c_upd = coh_upd*b*t_upd/sin(deg2rad(gamma));
    F_a_upd = rho_t*b*t_upd*v^2*sin(deg2rad(alpha))/sin(deg2rad(alpha+gamma));
    F_x_upd = m*g/Z_upd+(F_a_upd+F_c_upd)/(Z_upd*(sin(deg2rad(gamma))+tan(deg2rad(phi))*cos(deg2rad(gamma))));
    F_z_upd = F_x_upd*(cos(deg2rad(alpha))-mu*sin(deg2rad(alpha)))/(sin(deg2rad(alpha))+mu*cos(deg2rad(alpha)));
else
    F_x_upd = 0;
    F_z_upd = 0;
end

F_x = F_x*(B_tines-1)+F_x_upd;
F_z = F_z*(B_tines-1)+F_z_upd;

end

== matlab function eAgriBot_V4/Vehicle dynamics/Towed tool calculations/Tine forces/Front row ==
  data: phi input; tine_length input; tine_width input; rho_t input; mu input; c input; F_x output; angle input; tine_v_x input; depth input; F_z output; g input; F_tines input; h_upd input; coh_upd input
function [F_x, F_z] = fcn(phi, tine_length, tine_width, rho_t, mu, c, angle, tine_v_x, depth, g, F_tines, h_upd, coh_upd)

L_0 = tine_length;
b = tine_width;
alpha = rad2deg(angle);
t = -1*depth;
v = tine_v_x;

if t >= 0
    gamma = (90-phi)/2;
    t_e = t*sin(deg2rad(alpha+gamma))/sin(deg2rad(gamma));
    L_1 = t*cos(deg2rad(alpha+gamma))/sin(deg2rad(gamma));
    L_2 = t_e*tan(deg2rad(alpha));
    m = rho_t*t_e*b*(L_0+(L_1+L_2)/2);
    Z = (cos(deg2rad(gamma))-tan(deg2rad(phi))*sin(deg2rad(gamma)))/(sin(deg2rad(gamma))+tan(deg2rad(phi))*cos(deg2rad(gamma)))+...
        (cos(deg2rad(alpha))-mu*sin(deg2rad(alpha)))/(sin(deg2rad(alpha))+mu*cos(deg2rad(alpha)));
    F_c = c*b*t/sin(deg2rad(gamma));
    F_a = rho_t*b*t*v^2*sin(deg2rad(alpha))/sin(deg2rad(alpha+gamma));
    F_x = m*g/Z+(F_a+F_c)/(Z*(sin(deg2rad(gamma))+tan(deg2rad(phi))*cos(deg2rad(gamma))));
    F_z = F_x*(cos(deg2rad(alpha))-mu*sin(deg2rad(alpha)))/(sin(deg2rad(alpha))+mu*cos(deg2rad(alpha)));
else
    F_x = 0;
    F_z = 0;
end

% One tine is in the ruts left by the robot tires
t_upd = h_upd*(-1);
if t_upd >= 0
    gamma = (90-phi)/2;
    t_e_upd = t_upd*sin(deg2rad(alpha+gamma))/sin(deg2rad(gamma));
    L_1_upd = t_upd*cos(deg2rad(alpha+gamma))/sin(deg2rad(gamma));
    L_2_upd = t_e_upd*tan(deg2rad(alpha));
    m = rho_t*t_e_upd*b*(L_0+(L_1_upd+L_2_upd)/2);
    Z_upd = (cos(deg2rad(gamma))-tan(deg2rad(phi))*sin(deg2rad(gamma)))/(sin(deg2rad(gamma))+tan(deg2rad(phi))*cos(deg2rad(gamma)))+...
        (cos(deg2rad(alpha))-mu*sin(deg2rad(alpha)))/(sin(deg2rad(alpha))+mu*cos(deg2rad(alpha)));
    F_c_upd = coh_upd*b*t_upd/sin(deg2rad(gamma));
    F_a_upd = rho_t*b*t_upd*v^2*sin(deg2rad(alpha))/sin(deg2rad(alpha+gamma));
    F_x_upd = m*g/Z_upd+(F_a_upd+F_c_upd)/(Z_upd*(sin(deg2rad(gamma))+tan(deg2rad(phi))*cos(deg2rad(gamma))));
    F_z_upd = F_x_upd*(cos(deg2rad(alpha))-mu*sin(deg2rad(alpha)))/(sin(deg2rad(alpha))+mu*cos(deg2rad(alpha)));
else
    F_x_upd = 0;
    F_z_upd = 0;
end

F_x = F_x*(F_tines-1)+F_x_upd;
F_z = F_z*(F_tines-1)+F_z_upd;


end

== matlab function eAgriBot_V4/Vehicle dynamics/Position and velocity of the wheels (output values are for wheel bottom points)/MATLAB Function1 ==
  data: RT_x input; RT_z input; FT_x input; FT_sigma_x output; FT_z input; r_rear input; r_front input; F_sigma_anglef input; F_tau_anglef input; F_sigma_angler input; F_tau_angler input; FT_sigma_z output; FT_tau_x output; FT_tau_z output; RT_sigma_x output; RT_sigma_z output; RT_tau_x output; RT_tau_z output
function [FT_sigma_x, FT_sigma_z, FT_tau_x, FT_tau_z,...
    RT_sigma_x, RT_sigma_z, RT_tau_x, RT_tau_z] = fcn(RT_x, RT_z,...
    FT_x, FT_z, r_rear, r_front, F_sigma_anglef, F_tau_anglef,...
    F_sigma_angler, F_tau_angler)

    FT_sigma_x = FT_x+r_front*sin(F_sigma_anglef);
    FT_sigma_z = FT_z+r_front-r_front*cos(F_sigma_anglef);

    FT_tau_x = FT_x+r_front*sin(F_tau_anglef);
    FT_tau_z = FT_z+r_front-r_front*cos(F_tau_anglef);

    RT_sigma_x = RT_x+r_rear*sin(F_sigma_angler);
    RT_sigma_z = RT_z+r_rear-r_rear*cos(F_sigma_angler);

    RT_tau_x = RT_x+r_rear*sin(F_tau_angler);
    RT_tau_z = RT_z+r_rear-r_rear*cos(F_tau_angler);

end

== matlab function eAgriBot_V4/Vehicle dynamics/Towed tool calculations/Tire model (Harrow)/Tire force calc1 ==
  data: T output; v_ms input; s_d input; h input; t_params input; params2 input; F_sigma_z output; w_tire_pure input; F_sigma_x output; F_sigma_angle output; F_tau_z output; F_tau_x output; F_tau_angle output
function [T, F_sigma_z, F_sigma_x, F_sigma_angle, F_tau_z, F_tau_x, F_tau_angle]  = fcn(v_ms, s_d, h, t_params, params2, w_tire_pure)

    %%

% function [W, F_x, T] = ReeceFuncSim_V1(s_d, h, t_params, params2)
    c = t_params(1); % Pa
    k_c = t_params(2); % 34 default
    k_phi = t_params(3); % 49.68 default
    % n = 0.7;
    phi = t_params(4); % deg
    k_xy = t_params(5); % m
    gamma_s = t_params(6); % N/m^3
    
    R_u = t_params(7); % m (tire radius)
    w = t_params(8); % m (tire width)
    c_0 = t_params(9);
    c_1 = t_params(10);
    c_0f = t_params(11);
    c_1f = t_params(12);
    n_0 = t_params(13);
    n_1 = t_params(14);
    k_1 = t_params(15);
    k_2 = t_params(16);
    k_3 = t_params(17);
    
    exit_angle = params2(1);
    reso = params2(2); % Angle resolution, number of segments per one degree
    
    theta_m_max = params2(3); % Maximum percentage of theta_e allowed for theta_m
    % Allowing this to go too high may result in issues with some
    % calculations outputting complex numbers.
    
    s_d_tol = params2(4);
    
    po = params2(5);
    
    if h < 0
        % Start with defining the angles for theta
        % Then calculate the different values, e.g., sigma_n
        % for each angle.
        % The angle theta starts counter-clockwise from the
        % bottom of the tire (page 3 (267))
        theta_e = min(acos((R_u+max(h,-R_u))/R_u), deg2rad(89));
        theta_b = deg2rad(exit_angle);
        if s_d < -1*s_d_tol
            a = 1/(1+abs(s_d));
        
            d = tan(deg2rad(45)-deg2rad(phi/2));
            
            theta_m = min(2*atan(d./(-a-1)+sqrt(d^2./(-a-1).^2-(-a+1)./(-a-1))), theta_m_max*theta_e);
        elseif s_d >= -1*s_d_tol && s_d <= 0
            a = 1/(1+abs(s_d));
            d = tan(deg2rad(45)-deg2rad(phi/2));
            tm1 = min(2*atan(d./(-a-1)+sqrt(d^2./(-a-1).^2-(-a+1)./(-a-1))), theta_m_max*theta_e);
            tm2 = min((c_0+c_1*abs(s_d)), theta_m_max)*theta_e;
            ft = (1/(s_d_tol)*s_d+1)^po;
            theta_m = (1-ft)*tm1+ft*tm2;
        else
            theta_m = min((c_0+c_1*abs(s_d)), theta_m_max)*theta_e;
        end
        
        angles = linspace(theta_b,theta_e,ceil(rad2deg(theta_e-theta_b)*reso));
        
        l_p = (theta_e-theta_b)*R_u; % Contact arc length
        n = n_0+n_1*abs(s_d);
        b = min(w, l_p);
        
        sigma_n = zeros(length(angles),1);
        W_dtheta = zeros(length(angles),1);
        tau_max = zeros(length(angles),1);
        tau_x = zeros(length(angles),1);
        F_x_dtheta = zeros(length(angles),1);
        T_dtheta = zeros(length(angles),1);
        j_x = zeros(length(angles),1);
        K_v = zeros(length(angles),1);

        F_sigma_dx = zeros(length(angles),1);
        F_sigma_dz = zeros(length(angles),1);
        F_tau_dx = zeros(length(angles),1);
        F_tau_dz = zeros(length(angles),1);

        sigma_theta = zeros(length(angles),1);
        tau_theta = zeros(length(angles),1);
        
        for i = 1:length(angles)
            if angles(i) >= theta_m
                sigma_n(i,1) = (c*k_c+b*gamma_s*k_phi)*(R_u/b)^n*(cos(angles(i))-cos(theta_e))^n;
            else
                sigma_n(i,1) = (c*k_c+b*gamma_s*k_phi)*(R_u/b)^n...
                    *(cos(theta_e-((angles(i)-theta_b)/(theta_m-theta_b)*(theta_e-theta_m)))-cos(theta_e))^n;
            end
            sigma_theta(i,1) = angles(i)*sigma_n(i,1);

            tau_max(i,1) = c+sigma_n(i,1)*tan(deg2rad(phi));
        
            if s_d > 0
                j_x(i,1) = R_u*((theta_e-angles(i))-(1-s_d)*(sin(theta_e)-sin(angles(i))));
            elseif s_d >= -1*s_d_tol && s_d <= 0
                j_x1 = R_u*((theta_e-angles(i))-(1-s_d)*(sin(theta_e)-sin(angles(i))));
                a = 1/(1+abs(s_d));
                K_v(i,1) = a*(((1+abs(s_d))*(sin(theta_e)-sin(theta_m)))/(theta_e-theta_m)-1);
                if angles(i) >= theta_m
                    j_x2 = R_u*((theta_e-angles(i))*(1+K_v(i,1)*(1+abs(s_d)))-(1+abs(s_d))*(sin(theta_e)-sin(angles(i))));
                else
                    j_x2 = R_u*((theta_m-angles(i))-(1+abs(s_d))*(sin(theta_m)-sin(angles(i))));
                end
                ft = (1/(s_d_tol)*s_d+1)^po;
                j_x(i,1) = (1-ft)*j_x2+ft*j_x1;
            else
                a = 1/(1+abs(s_d));
                K_v(i,1) = a*(((1+abs(s_d))*(sin(theta_e)-sin(theta_m)))/(theta_e-theta_m)-1);
                if angles(i) >= theta_m
                    j_x(i,1) = R_u*((theta_e-angles(i))*(1+K_v(i,1)*(1+abs(s_d)))-(1+abs(s_d))*(sin(theta_e)-sin(angles(i))));
                else
                    j_x(i,1) = R_u*((theta_m-angles(i))-(1+abs(s_d))*(sin(theta_m)-sin(angles(i))));
                end
            end
        end
        
        for ii = 1:length(angles)
        
            tau_x(ii,1) = max(min(tau_max(ii,1)*(1-exp(-j_x(ii,1)/k_xy)), abs(tau_max(ii,1))), -1*abs(tau_max(ii,1)));
            tau_theta(ii,1) = angles(ii)*tau_x(ii,1);
        
            W_dtheta(ii,1) = R_u*(sigma_n(ii,1)*cos(angles(ii))+tau_x(ii,1)*sin(angles(ii)));
            F_x_dtheta(ii,1) = R_u*(tau_x(ii,1)*cos(angles(ii))-sigma_n(ii,1)*sin(angles(ii)));
            T_dtheta(ii, 1) = R_u^2*tau_x(ii,1);

            F_sigma_dz(ii,1) = R_u*sigma_n(ii,1)*cos(angles(ii));
            F_sigma_dx(ii,1) = -1*R_u*sigma_n(ii,1)*sin(angles(ii));

            F_tau_dz(ii,1) = R_u*tau_x(ii,1)*sin(angles(ii));
            F_tau_dx(ii,1) = R_u*tau_x(ii,1)*cos(angles(ii));
        end
        
%             W = w*trapz(angles, W_dtheta);
%             F_x = w*trapz(angles, F_x_dtheta);
            T = w*trapz(angles, T_dtheta);

            F_sigma_z = w*trapz(angles, F_sigma_dz);
            F_sigma_x = w*trapz(angles, F_sigma_dx);
            F_sigma_angle = atan(-1*F_sigma_x/F_sigma_z);
            F_tau_z = w*trapz(angles, F_tau_dz);
            F_tau_x = w*trapz(angles, F_tau_dx);
            F_tau_angle = atan(F_tau_z/F_tau_x);

            F_sigma_angle = max(theta_b, min(theta_e, F_sigma_angle));
            F_tau_angle = max(theta_b, min(theta_e, F_tau_angle));

            if v_ms < 0.3/3.6
                F_sigma_angle = max(0, v_ms)*F_sigma_angle*3.6/0.3;
                F_tau_angle = max(0, v_ms)*F_tau_angle*3.6/0.3;
            end
    else
%         W = 0;
%         F_x = 0;
        T = 0;

        F_sigma_z = 0;
        F_sigma_x = 0;
        F_sigma_angle = 0;
        F_tau_z = 0;
        F_tau_x = 0;
        F_tau_angle = 0;
    end

    %%
    
%     if v_ms <= v_low/3.6
%         F_t = (T_axle-J*a_ms/R_u)/R_u;
%         F_t_res = (T_axle-J*a_ms/R_u)/R_u;
%         P = P_lim;
%     elseif (v_ms > v_low/3.6) && (v_up <= 1/3.6)
%     %          F_t = 3.6*(1/(v_up-v_low))*(v_up/3.6-v_ms)*(T_axle-J*a_ms/r)/r+3.6*(1/(v_up-v_low))*(v_ms-v_low/3.6)*(F_z*mu-F_rr);
%          F_t = 3.6*(1/(v_up-v_low))*(v_up/3.6-v_ms)*(T_axle-J*a_ms/R_u)/R_u+3.6*(1/(v_up-v_low))*(v_ms-v_low/3.6)*(F_x);
%          F_t_res = 3.6*(1/(v_up-v_low))*(v_up/3.6-v_ms)*(T_axle-J*a_ms/R_u)/R_u+3.6*(1/(v_up-v_low))*(v_ms-v_low/3.6)*(T/R_u);
%          P = 3.6*(1/(v_up-v_low))*(v_up/3.6-v_ms)*P_lim;
%     else
%         F_t = F_x;
%         F_t_res = T/R_u;
%         P = 0;
%     end

%     F_t = F_x;
    if w_tire_pure <= 0 && v_ms <= 0
%         F_t = 0;
        F_sigma_x = 0;
        F_tau_x = 0;
    end
%     if v_ms <= 0
% %         F_t = max(0, F_t);
%         F_sigma_x = max(0, F_sigma_x);
%         F_tau_x = max(0, F_tau_x);
%     end
    if w_tire_pure <= 0
%         F_t = min(0, F_t);
        F_sigma_x = min(0, F_sigma_x);
        F_tau_x = min(0, F_tau_x);
    end
%     F_t_res = T/R_u;
%     P = 0;
%     P = min(max(P, 0), P_lim);
%     T_Ft_res = F_t_res*R_u+P*(w_tire-v_ms/R_u);
%     T_Ft = F_t*R_u;

    if v_ms < 0
%         F_sigma_x = max(100*abs(v_ms), F_sigma_x);
        F_tau_x = max(200*abs(v_ms), F_tau_x);
    end

    F_sigma_x = F_sigma_x*abs(tanh(20*v_ms));
    F_tau_x = F_tau_x*abs(tanh(20*v_ms));

%     if v_ms >= 0 && v_ms < 0.1/3.6 && w_tire_pure <= 0
% %         F_tau_x = F_tau_x-1e5*v_ms;
%         F_tau_x = -1e1*tanh(50*v_ms);
%         F_sigma_x = 0;
%     end

end

== matlab function eAgriBot_V4/Vehicle dynamics/Towed tool calculations/Tire model (Harrow)/slip_ratio calc ==
  data: r_har input; v_ms input; Har_tire_vx input; w_tire input; sr output; slip_ub_har input
function sr = fcn(r_har, v_ms, Har_tire_vx, w_tire, slip_ub_har)
    
    ub = slip_ub_har; % upper bound (when the rotational speed is 1 rad/s)
    lb = 0.1/3.6; % lower bound

    v_ms = max(0, v_ms);

    if abs(v_ms) > ub
        sr = (w_tire*r_har-Har_tire_vx)/Har_tire_vx;
    elseif abs(v_ms) < lb
        sr = w_tire*r_har-Har_tire_vx;
    elseif abs(v_ms) <= ub && abs(v_ms) >= lb
        sr = (1/(ub-lb))*(ub-v_ms)*(w_tire*r_har-Har_tire_vx)+(1/(ub-lb))*(v_ms-lb)*((w_tire*r_har-Har_tire_vx)/Har_tire_vx);
    else
        sr = 0;
    end

    sr = max(-1, sr);

end

== matlab function eAgriBot_V4/Vehicle dynamics/Towed tool calculations/Tire force positions/MATLAB Function1 ==
  data: Har_tire_x input; Har_tire_sigma_x output; Har_tire_z input; Har_tire_rad input; F_sigma_anglehar input; F_tau_anglehar input; Har_tire_sigma_z output; Har_tire_tau_x output; Har_tire_tau_z output
function [Har_tire_sigma_x, Har_tire_sigma_z, Har_tire_tau_x, Har_tire_tau_z] =...
    fcn(Har_tire_x, Har_tire_z, Har_tire_rad, F_sigma_anglehar, F_tau_anglehar)

    Har_tire_sigma_x = Har_tire_x+Har_tire_rad*sin(F_sigma_anglehar);
    Har_tire_sigma_z = Har_tire_z+Har_tire_rad-Har_tire_rad*cos(F_sigma_anglehar);

    Har_tire_tau_x = Har_tire_x+Har_tire_rad*sin(F_tau_anglehar);
    Har_tire_tau_z = Har_tire_z+Har_tire_rad-Har_tire_rad*cos(F_tau_anglehar);

end

== matlab function eAgriBot_V4/Vehicle dynamics/Ground properties update for tines/MATLAB Function ==
  data: t_params input; ground_res input; ground_height output; dens output; coh output; kx output; params2 input; FT_x input; FT_z input; sr_f input; ground_height input; dens input; coh input; kx input; prev_index input; index output
function [ground_height, dens, coh, kx, index]= fcn(t_params, ground_res, params2,...
    FT_x, FT_z, sr_f, ground_height, dens, coh, kx, prev_index)

    R_u = t_params(7);
    ea = deg2rad(params2(1));
    c = t_params(1);
    gamma_s = t_params(6);
    k_x = t_params(5);
    k_1 = t_params(15);
    k_2 = t_params(16);
    k_3 = t_params(17);

    n_p = 2;

    FT_exit_x = FT_x+R_u*sin(ea);
    FT_exit_z = FT_z+(R_u-R_u*cos(ea));

    FT_exit_dens = gamma_s*(1+(1-exp(-abs(sr_f)/k_1))*k_2+k_3*n_p);
    FT_exit_coh = c*(1+(1-exp(-abs(sr_f)/k_1))*k_2+k_3*n_p);
    FT_exit_kx = k_x*(1-(1-exp(-abs(sr_f)/k_1))*k_2-k_3*n_p);

    index = round(FT_exit_x/ground_res)+1;

    ground_height(index,1) = FT_exit_z;

    dens(index,1) = FT_exit_dens;

    coh(index,1) = FT_exit_coh;

    kx(index,1) = FT_exit_kx;

    if index > (prev_index+1)
        num_points_tofix = index-(prev_index+1);
        for i = 1:num_points_tofix
            ground_height(prev_index+i,1) = (ground_height(index,1)-ground_height(prev_index,1))*...
                i/(num_points_tofix+1)+ground_height(prev_index,1);

            dens(prev_index+i,1) = (dens(index,1)-dens(prev_index,1))*...
                i/(num_points_tofix+1)+dens(prev_index,1);

            coh(prev_index+i,1) = (coh(index,1)-coh(prev_index,1))*...
                i/(num_points_tofix+1)+coh(prev_index,1);

            kx(prev_index+i,1) = (kx(index,1)-kx(prev_index,1))*...
                i/(num_points_tofix+1)+kx(prev_index,1);
        end
    end

end

== matlab function eAgriBot_V4/Vehicle dynamics/Ground properties update for tines/MATLAB Function1 ==
  data: F_tine_x input; F_tine_z input; ground_height input; dens input; coh input; kx input; ground_res input; upd_F_tine_depth output; upd_dens output; upd_coh output; upd_kx output
function [upd_F_tine_depth, upd_dens, upd_coh, upd_kx] = fcn(F_tine_x, F_tine_z, ground_height, dens, coh, kx, ground_res)

    
    ind_L = max(floor((F_tine_x)/ground_res)+1, 1);
    ind_R = max(ceil((F_tine_x)/ground_res)+1, 1);

    upd_F_tine_depth = F_tine_z-mean(ground_height(ind_L:ind_R));
    upd_dens = mean(dens(ind_L:ind_R));
    upd_coh = mean(coh(ind_L:ind_R));
    upd_kx = mean(kx(ind_L:ind_R));

end
